simulink model "RocketSim"  (R2019b)
settings: Solver=VariableStepAuto  StartTime=0.0  StopTime=40  RelTol=1e-3
model workspace: external: MAT-File C:\Users\anshu\Desktop\Illinois_Space_Society\IREC_2021\RocketData.mat (data not in the file)
undefined symbols (not defined in the file): I, r
libraries: aerolibatmos2 x1, simulink x1
settings Model: OrderedModelArguments=off  Creator=anshu  LastModifiedBy=anshu

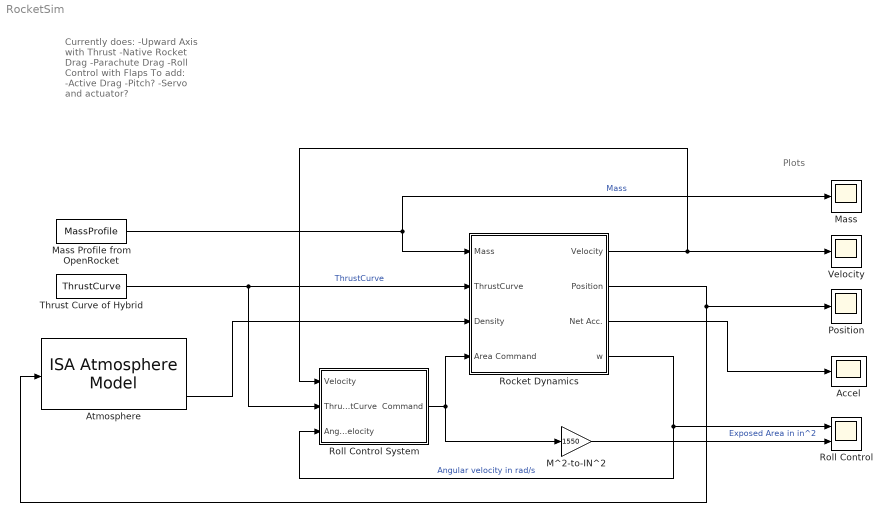
== system RocketSim ==
  note: Currently does:
      | -Upward Axis with Thrust
      | -Native Rocket Drag
      | -Parachute Drag
      | -Roll Control with Flaps
      |
      | To add:
      | -Active Drag
      | -Pitch?
      | -Servo and actuator?
  note: Plots
  Accel : Scope
  Atmosphere : aerolibatmos2/ISA Atmosphere Model  custom=off  g=9.80665  gamma=1.4  R=287.0531  L=0.0065  h_trop=11000  h_strat=20000  rho0=1.225  P0=101325  T0=288.15  h0=0
      settings: SourceProductName=Aerospace Blockset
  M^2-to-IN^2 : Gain  Gain=1550
  Mass : Scope
  Mass Profile from OpenRocket : FromWorkspace  VariableName=MassProfile  SampleTime=0  OutputAfterFinalValue=Holding final value
  Position : Scope
  Rocket Dynamics : Subsystem
  Roll Control : Scope  NumInputPorts=2
  Roll Control System : Subsystem
  "Thrust Curve of Hybrid " : FromWorkspace  VariableName=ThrustCurve  SampleTime=0  OutputAfterFinalValue=Holding final value
  Velocity : Scope
  wires:
  Rocket Dynamics/2(Position) -> Position/1, Atmosphere/1
  Atmosphere/4 -> Rocket Dynamics/3(Density)
  Rocket Dynamics/3(Net Acc.) -> Accel/1
  Rocket Dynamics/1(Velocity) -> Roll Control System/1(Velocity), Velocity/1
  Mass Profile from OpenRocket/1 -> Rocket Dynamics/1(Mass), Mass/1  "Mass"
  "Thrust Curve of Hybrid "/1 -> Rocket Dynamics/2(ThrustCurve), Roll Control System/2(ThrustCurve)  "ThrustCurve"
  Rocket Dynamics/4(w) -> Roll Control System/3(Angular Velocity), Roll Control/1  "Angular velocity in rad/s"
  M^2-to-IN^2/1 -> Roll Control/2  "Exposed Area in in^2"
  Roll Control System/1(Command) -> Rocket Dynamics/4(Area Command), M^2-to-IN^2/1

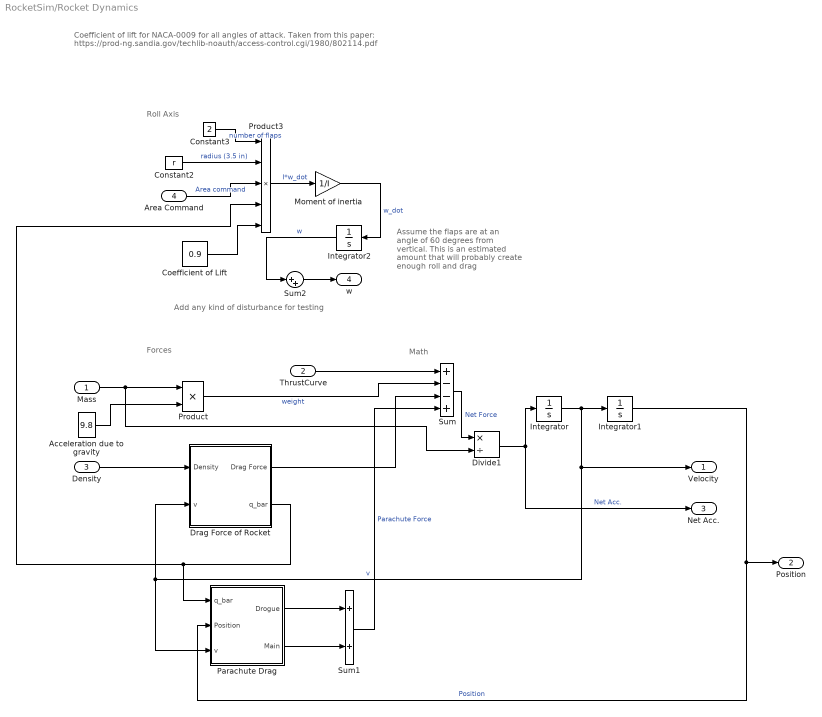
== system RocketSim/Rocket Dynamics ==
  note: Add any kind of disturbance for testing
  note: Coefficient of lift for NACA-0009 for all angles of attack. Taken from this paper:
      | https://prod-ng.sandia.gov/techlib-noauth/access-control.cgi/1980/802114.pdf
  note: Assume the flaps are at an angle of 60 degrees from vertical. This is an estimated amount that will probably create enough roll and drag
  note: Roll Axis
  note: Forces
  note: Math
  Mass : Inport
  ThrustCurve : Inport  Port=2
  Density : Inport  Port=3
  Area Command : Inport  Port=4
  Acceleration due to gravity : Constant  Value=9.8
  Coefficient of Lift : Constant  Value=0.9
  Constant2 : Constant  Value=r
  Constant3 : Constant  Value=2
  Divide1 : Product  Inputs=*/
  Drag Force of Rocket : Subsystem
  Integrator : Integrator  InitialCondition=.1
  Integrator1 : Integrator
  Integrator2 : Integrator  InitialCondition=4
  Moment of inertia : Gain  Gain=1/I
  Parachute Drag : Subsystem
  Product : Product
  Product3 : Product  Inputs=5
  Sum : Sum  Inputs=+--+
  Sum1 : Sum  Inputs=2
  Sum2 : Sum  Inputs=|++
  Velocity : Outport
  Position : Outport  Port=2
  Net Acc. : Outport  Port=3
  w : Outport  Port=4  VectorParamsAs1DForOutWhenUnconnected=off
  wires:
  Integrator1/1 -> Parachute Drag/2(Position), Position/1  "Position"
  Sum1/1 -> Sum/4  "Parachute Force"
  Divide1/1 -> Net Acc./1, Integrator/1  "Net Acc."
  Mass/1 -> Divide1/2, Product/1
  Sum/1 -> Divide1/1  "Net Force"
  Product/1 -> Sum/2  "weight"
  Acceleration due to gravity/1 -> Product/2
  ThrustCurve/1 -> Sum/1
  Integrator/1 -> Integrator1/1, Parachute Drag/3(v), Drag Force of Rocket/2(v), Velocity/1  "v"
  Area Command/1 -> Product3/3  "Area command"
  Constant3/1 -> Product3/1  "number of flaps"
  Product3/1 -> Moment of inertia/1  "I*w_dot"
  Constant2/1 -> Product3/2  "radius (3.5 in)"
  Moment of inertia/1 -> Integrator2/1  "w_dot"
  Coefficient of Lift/1 -> Product3/5
  Integrator2/1 -> Sum2/1  "w"
  ? -> Sum2/2
  Sum2/1 -> w/1
  Parachute Drag/1(Drogue) -> Sum1/1
  Parachute Drag/2(Main) -> Sum1/2
  Drag Force of Rocket/2(q_bar) -> Parachute Drag/1(q_bar), Product3/4
  Density/1 -> Drag Force of Rocket/1(Density)
  Drag Force of Rocket/1(Drag Force) -> Sum/3

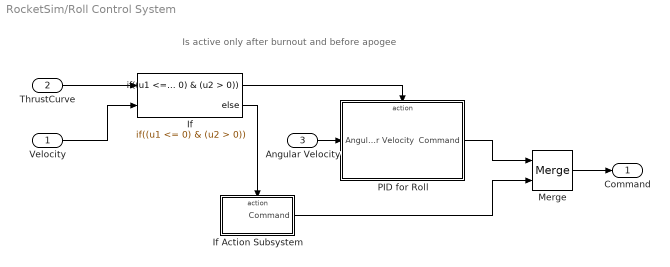
== system RocketSim/Roll Control System ==
  note: Is active only after burnout and before apogee
  Velocity : Inport
  ThrustCurve : Inport  Port=2
  Angular Velocity : Inport  Port=3
  If : If  NumInputs=2  IfExpression=(u1 <= 0) & (u2 > 0)
  If Action Subsystem : Subsystem  TreatAsAtomicUnit=on
  Merge : Merge
  PID for Roll : Subsystem  TreatAsAtomicUnit=on
  Command : Outport
  wires:
  If Action Subsystem/1(Command) -> Merge/2
  If/1 -> PID for Roll/Action
  ThrustCurve/1 -> If/1
  PID for Roll/1(Command) -> Merge/1
  If/2 -> If Action Subsystem/Action
  Angular Velocity/1 -> PID for Roll/1(Angular Velocity)
  Velocity/1 -> If/2
  Merge/1 -> Command/1

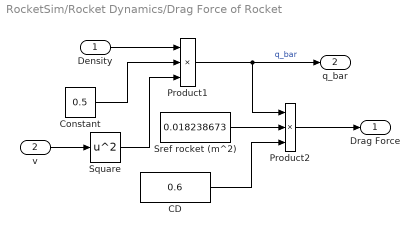
== system RocketSim/Rocket Dynamics/Drag Force of Rocket ==
  Density : Inport
  v : Inport  Port=2
  CD : Constant  Value=0.6
  Constant : Constant  Value=0.5
  Product1 : Product  Inputs=3
  Product2 : Product  Inputs=3
  Square : Math  Operator=square  SignedPower=off  SaturateOnIntegerOverflow=on
  Sref rocket (m^2) : Constant  Value=0.018238673
  Drag Force : Outport
  q_bar : Outport  Port=2
  wires:
  Density/1 -> Product1/1
  Square/1 -> Product1/3
  v/1 -> Square/1
  Product2/1 -> Drag Force/1
  Constant/1 -> Product1/2
  Product1/1 -> q_bar/1, Product2/1  "q_bar"
  Sref rocket (m^2)/1 -> Product2/2
  CD/1 -> Product2/3

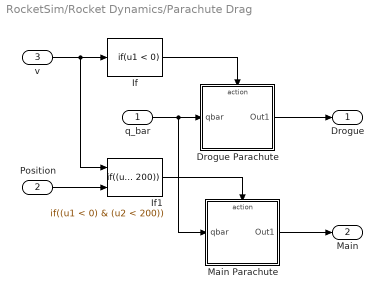
== system RocketSim/Rocket Dynamics/Parachute Drag ==
  q_bar : Inport
  Position : Inport  Port=2
  v : Inport  Port=3
  Drogue Parachute : Subsystem  TreatAsAtomicUnit=on
  If : If  IfExpression=u1 < 0  ShowElse=off
  If1 : If  NumInputs=2  IfExpression=(u1 < 0) & (u2 < 200)  ShowElse=off
  Main Parachute : Subsystem  TreatAsAtomicUnit=on
  Drogue : Outport
  Main : Outport  Port=2
  wires:
  q_bar/1 -> Main Parachute/1(qbar), Drogue Parachute/1(qbar)
  Main Parachute/1(Out1) -> Main/1
  If/1 -> Drogue Parachute/Action
  v/1 -> If1/1, If/1
  Position/1 -> If1/2
  If1/1 -> Main Parachute/Action
  Drogue Parachute/1(Out1) -> Drogue/1

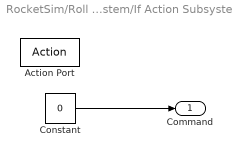
== system RocketSim/Roll Control System/If Action Subsystem ==
  Action Port : ActionPort  ActionPortLabel=else
  Constant : Constant  Value=0
  Command : Outport
  wires:
  Constant/1 -> Command/1

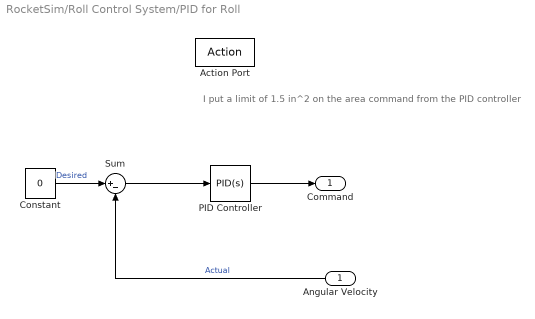
== system RocketSim/Roll Control System/PID for Roll ==
  note: I put a limit of 1.5 in^2 on the area command from the PID controller
  Angular Velocity : Inport
  Action Port : ActionPort  ActionPortLabel=if((u1 <= 0) & (u2 > 0))
  Constant : Constant  Value=0
  PID Controller : simulink/Continuous/PID Controller  Controller=PID  Form=Parallel  TimeDomain=Continuous-time  SampleTime=-1  IntegratorMethod=Forward Euler  FilterMethod=Forward Euler  ControllerParametersSource=internal  P=0.002  I=0.0015  D=0.001  UseFilter=on  N=1  TunerSelectOption=Frequency Response Based  InitialConditionSource=internal  InitialConditionForIntegrator=0  InitialConditionForFilter=0  DifferentiatorICPrevScaledInput=0  ExternalReset=none  TrackingMode=off  Kt=1  LimitOutput=on  UpperSaturationLimit=0.00096774  LowerSaturationLimit=-0.00096774  LinearizeAsGain=off  AntiWindupMode=none  Kb=1  POutMin=[]  POutMax=[]  IOutMin=[]  IOutMax=[]  DOutMin=[]  DOutMax=[]  NOutMin=[]  NOutMax=[]  SumOutMin=[]  SumOutMax=[]  SaturationOutMin=[]  SaturationOutMax=[]  PParamMin=[]  PParamMax=[]  IParamMin=[]  IParamMax=[]  DParamMin=[]  DParamMax=[]  NParamMin=[]  NParamMax=[]  KbParamMin=[]  KbParamMax=[]  KtParamMin=[]  KtParamMax=[]  KbOutMin=[]  KbOutMax=[]  KtOutMin=[]  KtOutMax=[]  IntegratorOutMin=[]  IntegratorOutMax=[]  FilterOutMin=[]  FilterOutMax=[]  SumI1OutMin=[]  SumI1OutMax=[]  SumI2OutMin=[]  SumI2OutMax=[]  SumI3OutMin=[]  SumI3OutMax=[]  SumI4OutMin=[]  SumI4OutMax=[]  SumDOutMin=[]  SumDOutMax=[]  DifferentiatorOutMin=[]  DifferentiatorOutMax=[]  FilterDiffOutCoefMin=[]  FilterDiffOutCoefMax=[]  ReciprocalOutMin=[]  ReciprocalOutMax=[]  SumDenOutMin=[]  SumDenOutMax=[]  SumNumOutMin=[]  SumNumOutMax=[]  DivideOutMin=[]  DivideOutMax=[]  IntegratorContinuousStateAttributes=''  IntegratorStateMustResolveToSignalObject=off  IntegratorRTWStateStorageClass=Auto  FilterContinuousStateAttributes=''  FilterStateMustResolveToSignalObject=off  FilterRTWStateStorageClass=Auto  ParallelPVariant=InternalParameters  IdealPVariant=Disabled  IVariant=InternalParameters  DVariant=InternalParameters  IntegratorVariant=Continuous  SatVariant=Enabled  AWVariant=Passthrough  PCopyVariant=Disabled  TRVariant=Disabled  FdbkBlocksVariant=Forward  IdealPFdbkVariant=Disabled  SatFdbkVariant=Disabled  DerivativeFilterVariant=ContFilter  NVariant=InternalParameters  NCopyVariant=Disabled  FilterICVariant=InternalICsFilter  IntegratorICVariant=InternalICs  ExternalResetVariant=Disabled  TRSumVariant=Passthrough  SumFdbkVariant=Disabled  SumVariant=Sum_PID
  Sum : Sum  Inputs=|+-
  Command : Outport
  wires:
  Angular Velocity/1 -> Sum/2  "Actual"
  Constant/1 -> Sum/1  "Desired"
  PID Controller/1 -> Command/1
  Sum/1 -> PID Controller/1

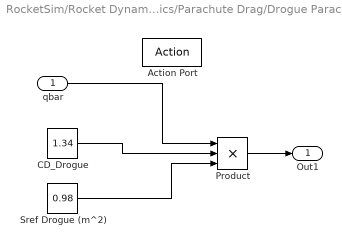
== system RocketSim/Rocket Dynamics/Parachute Drag/Drogue Parachute ==
  qbar : Inport
  Action Port : ActionPort  ActionPortLabel=if(u1 < 0)
  CD_Drogue : Constant  Value=1.34
  Product : Product  Inputs=3
  Sref Drogue (m^2) : Constant  Value=0.98
  Out1 : Outport
  wires:
  qbar/1 -> Product/1
  CD_Drogue/1 -> Product/2
  Sref Drogue (m^2)/1 -> Product/3
  Product/1 -> Out1/1

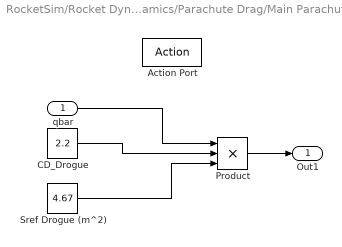
== system RocketSim/Rocket Dynamics/Parachute Drag/Main Parachute ==
  qbar : Inport
  Action Port : ActionPort  ActionPortLabel=if((u1 < 0) & (u2 < 200))
  CD_Drogue : Constant  Value=2.2
  Product : Product  Inputs=3
  Sref Drogue (m^2) : Constant  Value=4.67
  Out1 : Outport
  wires:
  qbar/1 -> Product/1
  CD_Drogue/1 -> Product/2
  Sref Drogue (m^2)/1 -> Product/3
  Product/1 -> Out1/1
